simulink model "Second Exercise"  (R2017a)
settings: Solver=VariableStepAuto  StartTime=0.0  StopTime=500  RelTol=1e-3
undefined symbols (not defined in the file): Afs, As, Cw, g, m, p
libraries: simulink x1
settings Model: Creator=18181  LastModifiedBy=18181

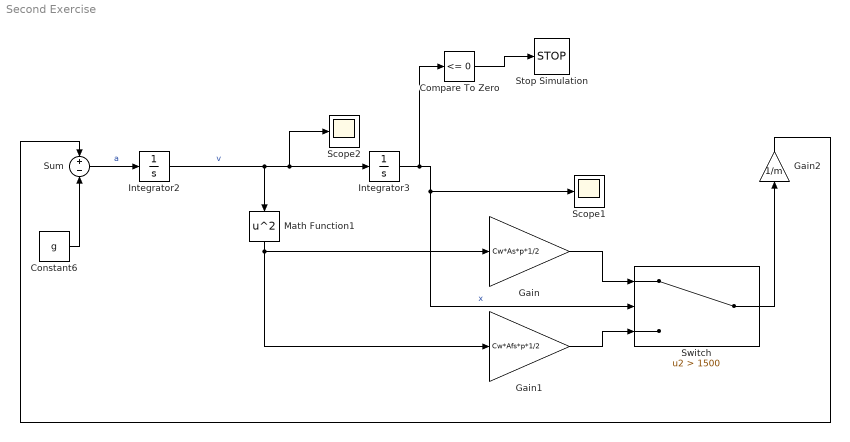
== system Second Exercise ==
  Compare To Zero : simulink/Logic and Bit Operations/Compare To Zero  relop=<=  OutDataTypeStr=boolean
  Constant6 : Constant  Value=g
  Gain : Gain  Gain=Cw*As*p*1/2
  Gain1 : Gain  Gain=Cw*Afs*p*1/2
  Gain2 : Gain  Gain=1/m
  Integrator2 : Integrator
  Integrator3 : Integrator  InitialCondition=3000
  Math Function1 : Math  Operator=square  SaturateOnIntegerOverflow=on
  Scope1 : Scope
  Scope2 : Scope
  Stop Simulation : Stop
  Sum : Sum  Inputs=+-
  Switch : Switch  Criteria=u2 > Threshold  Threshold=1500
  wires:
  Integrator2/1 -> Math Function1/1, Scope2/1, Integrator3/1  "v"
  Integrator3/1 -> Compare To Zero/1, Switch/2, Scope1/1  "x"
  Constant6/1 -> Sum/2
  Sum/1 -> Integrator2/1  "a"
  Math Function1/1 -> Gain/1, Gain1/1
  Gain/1 -> Switch/1
  Gain1/1 -> Switch/3
  Switch/1 -> Gain2/1
  Gain2/1 -> Sum/1
  Compare To Zero/1 -> Stop Simulation/1
